simulink model "Differential_CS9"  (Simulink 8.8)
settings: Solver=ode45  StartTime=0  StopTime=100  FixedStep=0.002  RelTol=1e-3  AbsTol=1e-6
libraries: Solver_SF x1
settings Model: Creator=ywata  LastModifiedBy=mkhan  ExtModeTrigMode=oneshot  ExtModeArmWhenConnect=off
settings DataIOCC: LimitDataPoints=off  SignalLoggingName=sigsOut
settings OptimizationCC: BooleanDataType=off  ExpressionDepthLimit=2147483647
settings DebuggingCC: SaveWithParameterizedLinksMsg=none  SignalResolutionControl=TryResolveAllWithWarning  MultiTaskDSMMsg=warning  MultiTaskCondExecSysMsg=none  SFExecutionAtInitializationDiag=warning
settings HardwareCC: TargetUnknown=on
settings RTWCC: TemplateMakefile=grt_vc.tmf
settings ConfigComp: CovSFcnEnable=off

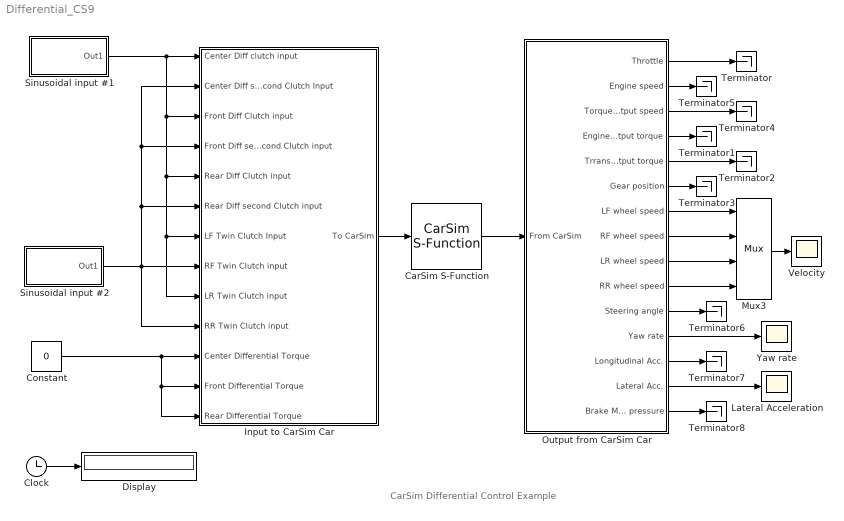
== system Differential_CS9 ==
  note: CarSim Differential Control Example
  CarSim S-Function : Solver_SF/CarSim S-Function  Priority=1  SIMFILE=simfile.sim  Run_RTs=off  vs_state_ind=Run  StopMode_ind=Vehicle Model
  Clock : Clock
  Constant : Constant  Value=0
  Display : Display
      settings: Format=bank  Decimation=100
  Input to CarSim Car : Subsystem
  Lateral Acceleration : Scope
  Mux3 : Mux
  Output from CarSim Car : Subsystem
  Sinusoidal input #1 : Subsystem
  Sinusoidal input #2 : Subsystem
  Terminator{,1..8} (9 alike) : Terminator
  Velocity : Scope
  Yaw rate : Scope
  wires:
  Sinusoidal input #1/1(Out1) -> Input to CarSim Car/1(Center Diff clutch input), Input to CarSim Car/3(Front Diff Clutch input), Input to CarSim Car/5(Rear Diff Clutch input), Input to CarSim Car/7(LF Twin Clutch Input), Input to CarSim Car/9(LR Twin Clutch input)
  Constant/1 -> Input to CarSim Car/11(Center Differential Torque), Input to CarSim Car/12("Front Differential Torque "), Input to CarSim Car/13(Rear Differential Torque)
  Mux3/1 -> Velocity/1
  Output from CarSim Car/7(LF wheel speed) -> Mux3/1
  Output from CarSim Car/8(RF wheel speed) -> Mux3/2
  Output from CarSim Car/9(LR wheel speed) -> Mux3/3
  Output from CarSim Car/10(RR wheel speed) -> Mux3/4
  Output from CarSim Car/12(Yaw rate) -> Yaw rate/1
  Output from CarSim Car/14(Lateral Acc.) -> Lateral Acceleration/1
  Output from CarSim Car/1(Throttle) -> Terminator/1
  Output from CarSim Car/4(Engine output torque) -> Terminator1/1
  Output from CarSim Car/5(Trransmission output torque) -> Terminator2/1
  Output from CarSim Car/6(Gear position) -> Terminator3/1
  Output from CarSim Car/3(Torque converter output speed) -> Terminator4/1
  Output from CarSim Car/2(Engine speed) -> Terminator5/1
  Output from CarSim Car/11(Steering angle) -> Terminator6/1
  Output from CarSim Car/13(Longitudinal Acc.) -> Terminator7/1
  Output from CarSim Car/15(Brake M/C pressure) -> Terminator8/1
  Sinusoidal input #2/1(Out1) -> Input to CarSim Car/8(RF Twin Clutch input), Input to CarSim Car/6(Rear Diff second Clutch input), Input to CarSim Car/4(Front Diff second Clutch input), Input to CarSim Car/2(Center Diff second Clutch Input), Input to CarSim Car/10(RR Twin Clutch input)
  CarSim S-Function/1 -> Output from CarSim Car/1(From CarSim)
  Input to CarSim Car/1(To CarSim) -> CarSim S-Function/1
  Clock/1 -> Display/1

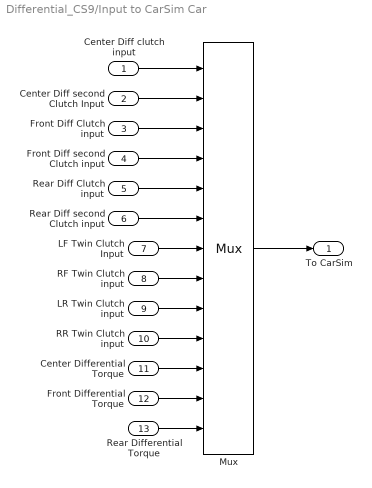
== system Differential_CS9/Input to CarSim Car ==
  Center Diff clutch input : Inport
  Center Diff second Clutch Input : Inport  Port=2
  Front Diff Clutch input : Inport  Port=3
  Front Diff second Clutch input : Inport  Port=4
  Rear Diff Clutch input : Inport  Port=5
  Rear Diff second Clutch input : Inport  Port=6
  LF Twin Clutch Input : Inport  Port=7
  RF Twin Clutch input : Inport  Port=8
  LR Twin Clutch input : Inport  Port=9
  RR Twin Clutch input : Inport  Port=10
  Center Differential Torque : Inport  Port=11
  "Front Differential Torque " : Inport  Port=12
  Rear Differential Torque : Inport  Port=13
  Mux : Mux  Inputs=13
  To CarSim : Outport
  wires:
  Mux/1 -> To CarSim/1
  Center Differential Torque/1 -> Mux/11
  Rear Differential Torque/1 -> Mux/13
  "Front Differential Torque "/1 -> Mux/12
  RR Twin Clutch input/1 -> Mux/10
  LR Twin Clutch input/1 -> Mux/9
  RF Twin Clutch input/1 -> Mux/8
  LF Twin Clutch Input/1 -> Mux/7
  Rear Diff second Clutch input/1 -> Mux/6
  Rear Diff Clutch input/1 -> Mux/5
  Front Diff second Clutch input/1 -> Mux/4
  Front Diff Clutch input/1 -> Mux/3
  Center Diff second Clutch Input/1 -> Mux/2
  Center Diff clutch input/1 -> Mux/1

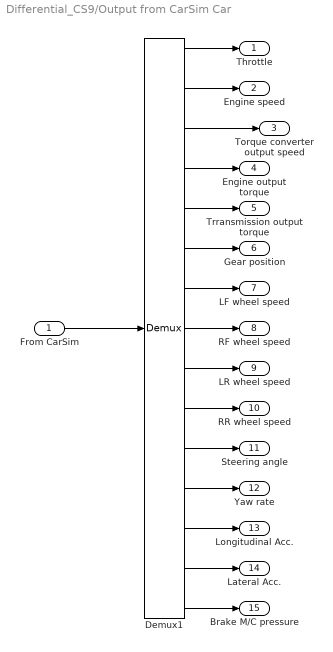
== system Differential_CS9/Output from CarSim Car ==
  From CarSim : Inport
  Demux1 : Demux  Outputs=15
      settings: DisplayOption=none
  Throttle : Outport
  Engine speed : Outport  Port=2
  Torque converter output speed : Outport  Port=3
  Engine output torque : Outport  Port=4
  Trransmission output torque : Outport  Port=5
  Gear position : Outport  Port=6
  LF wheel speed : Outport  Port=7
  RF wheel speed : Outport  Port=8
  LR wheel speed : Outport  Port=9
  RR wheel speed : Outport  Port=10
  Steering angle : Outport  Port=11
  Yaw rate : Outport  Port=12
  Longitudinal Acc. : Outport  Port=13
  Lateral Acc. : Outport  Port=14
  Brake M/C pressure : Outport  Port=15
  wires:
  From CarSim/1 -> Demux1/1
  Demux1/1 -> Throttle/1
  Demux1/2 -> Engine speed/1
  Demux1/3 -> Torque converter output speed/1
  Demux1/7 -> LF wheel speed/1
  Demux1/13 -> Longitudinal Acc./1
  Demux1/14 -> Lateral Acc./1
  Demux1/15 -> Brake M/C pressure/1
  Demux1/8 -> RF wheel speed/1
  Demux1/9 -> LR wheel speed/1
  Demux1/10 -> RR wheel speed/1
  Demux1/11 -> Steering angle/1
  Demux1/12 -> Yaw rate/1
  Demux1/4 -> Engine output torque/1
  Demux1/5 -> Trransmission output torque/1
  Demux1/6 -> Gear position/1

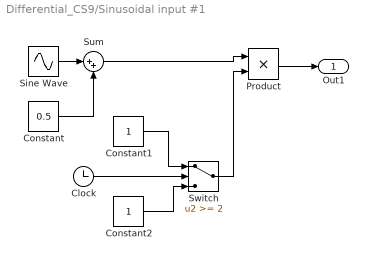
== system Differential_CS9/Sinusoidal input #1 ==
  Clock : Clock
  Constant : Constant  Value=0.5
  Constant1 : Constant
  Constant2 : Constant
  Product : Product  InputSameDT=on  SaturateOnIntegerOverflow=on  OutDataTypeStr=Inherit: Same as first input
  Sine Wave : Sin  Amplitude=0.5  Frequency=0.25*2*pi  Phase=3/2*pi  SampleTime=0
  Sum : Sum  Inputs=|++  InputSameDT=on  SaturateOnIntegerOverflow=on  OutDataTypeStr=Inherit: Same as first input
  Switch : Switch  Threshold=2  SaturateOnIntegerOverflow=on  InputSameDT=on
  Out1 : Outport
  wires:
  Sine Wave/1 -> Sum/1
  Constant/1 -> Sum/2
  Clock/1 -> Switch/2
  Constant1/1 -> Switch/1
  Constant2/1 -> Switch/3
  Switch/1 -> Product/2
  Product/1 -> Out1/1
  Sum/1 -> Product/1

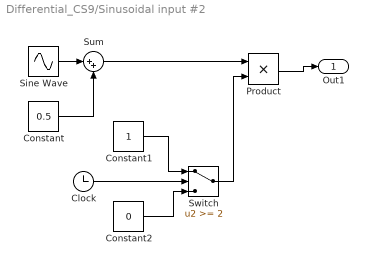
== system Differential_CS9/Sinusoidal input #2 ==
  Clock : Clock
  Constant : Constant  Value=0.5
  Constant1 : Constant
  Constant2 : Constant  Value=0
  Product : Product  InputSameDT=on  SaturateOnIntegerOverflow=on  OutDataTypeStr=Inherit: Same as first input
  Sine Wave : Sin  Amplitude=0.5  Frequency=0.25*2*pi  Phase=1/2*pi  SampleTime=0
  Sum : Sum  Inputs=|++  InputSameDT=on  SaturateOnIntegerOverflow=on  OutDataTypeStr=Inherit: Same as first input
  Switch : Switch  Threshold=2  SaturateOnIntegerOverflow=on  InputSameDT=on
  Out1 : Outport
  wires:
  Sine Wave/1 -> Sum/1
  Constant/1 -> Sum/2
  Clock/1 -> Switch/2
  Sum/1 -> Product/1
  Constant1/1 -> Switch/1
  Constant2/1 -> Switch/3
  Switch/1 -> Product/2
  Product/1 -> Out1/1
